simulink model "m020_Relay"  (R2022a)
settings: Solver=VariableStepAuto  StartTime=0.0  StopTime=10.0  RelTol=1e-3
model workspace (MAT data in the model file):
  HighLimit = 118
  LowLimit = 82
settings Model: Creator=Admin  LastModifiedBy=Admin

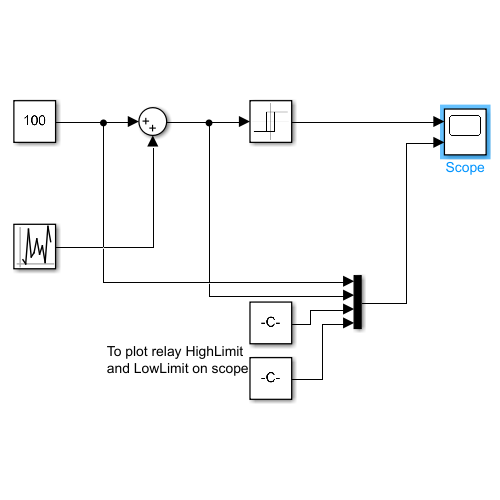
[thumbnail: Simulink's stored preview of the top-level diagram]
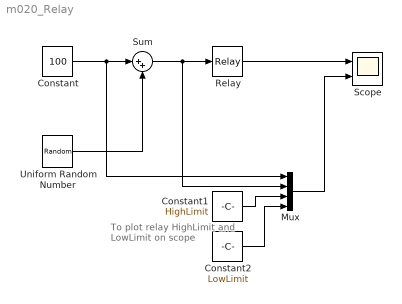
== system m020_Relay ==
  note: To plot relay HighLimit
      | and LowLimit on scope
  Constant : Constant  Value=100
  Constant1 : Constant  Value=HighLimit
  Constant2 : Constant  Value=LowLimit
  Mux : Mux
  Relay : Relay  OnSwitchValue=HighLimit  OffSwitchValue=LowLimit
  Scope : Scope  NumInputPorts=2
  Sum : Sum  Inputs=|++
  Uniform Random Number : UniformRandomNumber  Minimum=-20  Maximum=20  Seed=round(rand()*1000,0)  SampleTime=0.02
  wires:
  Uniform Random Number/1 -> Sum/2
  Sum/1 -> Mux/2, Relay/1
  Relay/1 -> Scope/1
  Constant/1 -> Mux/1, Sum/1
  Mux/1 -> Scope/2
  Constant1/1 -> Mux/3
  Constant2/1 -> Mux/4
